simulink model "Vadim"  (R2022a)
settings: Solver=FixedStepDiscrete  StartTime=0.0  StopTime=Time*9360  RelTol=1e-3
InitFcn:
  | Time = 40;
  | PowerDelay = Time*100;
values from neighbouring files (symbols this model uses):
  a = 0.0001    [Vadim.m]
  alpha = 0.4    [Vadim.m]
  R = 10    [Vadim.m]
libraries: sim_stud_lib_r2022a x5, dspsrcs4 x2, dspsigops x2, dspswit3 x1
settings Model: Creator=RolePups  LastModifiedBy=RolePups

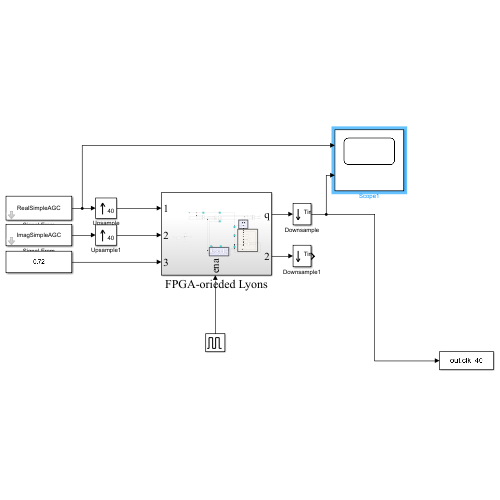
[thumbnail: Simulink's stored preview of the top-level diagram]
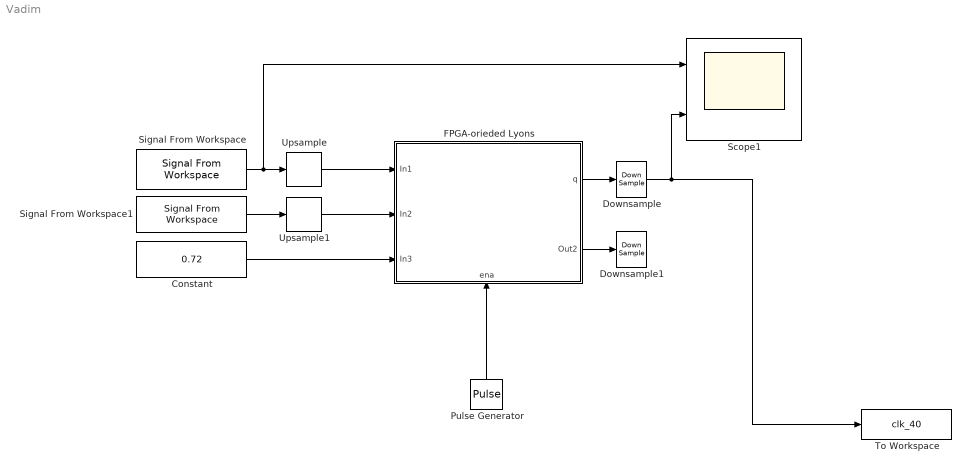
== system Vadim ==
  Constant : Constant  Value=0.72
  Downsample : DownSample  N=Time  RateOptions=Allow multirate processing
  Downsample1 : DownSample  N=Time  RateOptions=Allow multirate processing
  FPGA-orieded Lyons : Subsystem
      settings: PortSchema="{\"entries\":[{\"content\":{\"sides\":[{\"content\":{\"connectorIds\":[\"In1\",\"In2\",\"In3\"]},\"type\":\"ConnectorPlacement.EquallySpacedRectSide\",\"uuid\":\"2382ef4f-8b23-4fd9-9999-ae4ff3838c30\"},{\"content\":{\"connectorIds\":[\"Out1\",\"Out2\"],\"side\":\"RIGHT\"},\"type\":\"ConnectorPlacement.EquallySpacedRectSide\",\"uuid\":\"ff744322-ad90-46d9-948c-0637f52c7b9c\"},{\"content\":{\"connectorIds\":[],\"side\":\"TOP\"},\"type\":\"ConnectorPlacement.EquallySpacedRectSide\",\"uuid\":\"b0276f26-9e78-4e39-abf6-7a1348b88309\"},{\"content\":{\"connectorIds\":[\"In4\"],\"side\":\"BOTTOM\"},\"type\":\"ConnectorPlacement.EquallySpacedRectSide\",\"uuid\":\"b0dd70ff-8907-4b14-a46e-e3bbf4bdcae4\"}]},\"type\":\"ConnectorPlacement.EquallySpacedConnector\",\"uuid\":\"3f5cde89-4d4f-4bf7-b554-70cc79020603\"}],\"packageUris\":[\"http://schema.mathworks.com/mf0/Connector/R2020b\"],\"version\":\"1.0\"}"
  Pulse Generator : DiscretePulseGenerator  PulseType=Time based  Period=Time  PulseWidth=1/Time*100
  Scope1 : Scope  NumInputPorts=2
  Signal From Workspace : dspsrcs4/Signal From Workspace  X=RealSimpleAGC  Ts=Time  nsamps=1  OutputAfterFinalValue=Setting to zero  ignoreOrWarnInputAndFrameLengths=off  OutputFrames=off
  Signal From Workspace1 : dspsrcs4/Signal From Workspace  X=ImagSimpleAGC  Ts=Time  nsamps=1  OutputAfterFinalValue=Setting to zero  ignoreOrWarnInputAndFrameLengths=off  OutputFrames=off
  To Workspace : ToWorkspace  VariableName=clk_40  SampleTime=-1
  Upsample : dspsigops/Upsample  N=Time  phase=0  RateOptions=Allow multirate processing  ic=0  mode=Unused parameter value
  Upsample1 : dspsigops/Upsample  N=Time  phase=0  RateOptions=Allow multirate processing  ic=0  mode=Unused parameter value
  wires:
  Signal From Workspace/1 -> Scope1/1, Upsample/1
  Signal From Workspace1/1 -> Upsample1/1
  Upsample1/1 -> FPGA-orieded Lyons/2(In2)
  Constant/1 -> FPGA-orieded Lyons/3(In3)
  Pulse Generator/1 -> FPGA-orieded Lyons/4(ena)
  Upsample/1 -> FPGA-orieded Lyons/1(In1)
  FPGA-orieded Lyons/1(q) -> Downsample/1
  Downsample/1 -> Scope1/2, To Workspace/1
  FPGA-orieded Lyons/2(Out2) -> Downsample1/1

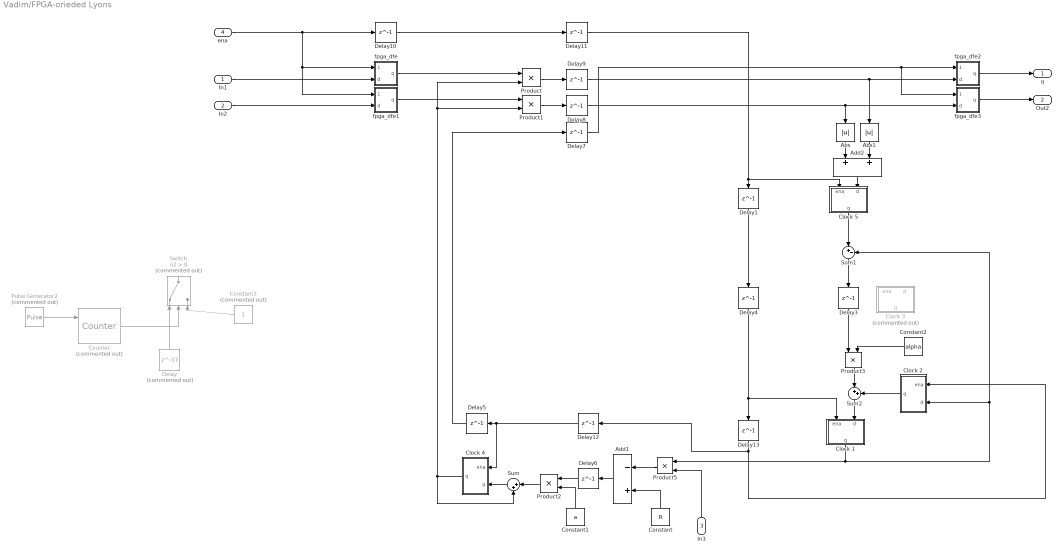
== system Vadim/FPGA-orieded Lyons ==
  In1 : Inport
  In2 : Inport  Port=2
  In3 : Inport  Port=3
  ena : Inport  Port=4
  Abs : Abs  SaturateOnIntegerOverflow=off
  Abs1 : Abs  SaturateOnIntegerOverflow=off
  Add1 : Sum  Inputs=-+  AccumDataTypeStr=double
  Add2 : Sum  AccumDataTypeStr=double
  Clock 1 : Subsystem
  Clock 2 : Subsystem
  Clock 3 : Subsystem  Commented=on
  Clock 4 : Subsystem
  Clock 5 : Subsystem
  Constant : Constant  Value=R  SampleTime=-1
  Constant1 : Constant  Value=a  SampleTime=-1
  Constant2 : Constant  Value=alpha  SampleTime=-1
  Constant3 : Constant  Commented=on  SampleTime=-1
  Counter : dspswit3/Counter  Commented=on  Direction=Up  CountEvent=Rising edge  CounterSize=User defined  MaxCount=1  InitialCount=0  Output=Count  HitValue=32  ResetInput=on  SamplesPerFrame=1  Ts=1  CntDtype=double  HitDtype=Logical
  Delay : Delay  Commented=on  DelayLength=37  InitialCondition=0
  Delay{1,3..13} (12 alike) : Delay  DelayLength=1  InitialCondition=0
  Product{,1..3,5} (5 alike) : Product  OutDataTypeStr=double
  Pulse Generator2 : DiscretePulseGenerator  Commented=on  PulseType=Time based  Period=Time*20000  PulseWidth=50  PhaseDelay=41
  Sum : Sum  Inputs=|++  AccumDataTypeStr=double
  Sum1 : Sum  Inputs=|+-  AccumDataTypeStr=double
  Sum2 : Sum  Inputs=|++  AccumDataTypeStr=double
  Switch : Switch  Commented=on  Criteria=u2 > Threshold  SaturateOnIntegerOverflow=off  InputSameDT=off
  fpga_dfe : Subsystem  AncestorBlock=sim_stud_lib_r2022a/fpga_dfe
      mask Display:
      | disp('D');
      | port_label('input',1,'e');
      | port_label('input',2,'d');
      | port_label('output',1,'q');
  fpga_dfe1 : Subsystem  AncestorBlock=sim_stud_lib_r2022a/fpga_dfe
      mask Display:
      | disp('D');
      | port_label('input',1,'e');
      | port_label('input',2,'d');
      | port_label('output',1,'q');
  fpga_dfe2 : Subsystem  AncestorBlock=sim_stud_lib_r2022a/fpga_dfe
      mask Display:
      | disp('D');
      | port_label('input',1,'e');
      | port_label('input',2,'d');
      | port_label('output',1,'q');
  fpga_dfe3 : Subsystem  AncestorBlock=sim_stud_lib_r2022a/fpga_dfe
      mask Display:
      | disp('D');
      | port_label('input',1,'e');
      | port_label('input',2,'d');
      | port_label('output',1,'q');
  q : Outport
  Out2 : Outport  Port=2
  wires:
  Clock 4/1(q) -> Sum/2, Product1/2, Product/2
  Product/1 -> Delay9/1
  Product1/1 -> Delay8/1
  Constant/1 -> Add1/2
  Sum/1 -> Clock 4/2(d)
  Product2/1 -> Sum/1
  Constant1/1 -> Product2/2
  Abs1/1 -> Add2/2
  Abs/1 -> Add2/1
  In3/1 -> Product5/2
  Product5/1 -> Add1/1
  Constant2/1 -> Product3/2
  Product3/1 -> Sum2/1
  Clock 2/1(q) -> Sum2/2
  fpga_dfe/1(q) -> Product/1
  fpga_dfe1/1(q) -> Product1/1
  Add1/1 -> Delay6/1
  Constant3/1 -> Switch/3
  Counter/1 -> Switch/2
  Pulse Generator2/1 -> Counter/1
  Sum2/1 -> Clock 1/2(d)
  Clock 1/1(q) -> Product5/1, Sum1/2, Clock 2/2(d)
  Delay/1 -> Switch/1
  fpga_dfe2/1(q) -> q/1
  fpga_dfe3/1(q) -> Out2/1
  Add2/1 -> Clock 5/2(d)
  Clock 5/1(q) -> Sum1/1
  In1/1 -> fpga_dfe/2(d)
  In2/1 -> fpga_dfe1/2(d)
  Delay8/1 -> fpga_dfe3/2(d), Abs/1
  Delay9/1 -> Abs1/1, fpga_dfe2/2(d)
  Sum1/1 -> Delay3/1
  Delay3/1 -> Product3/1
  Delay4/1 -> Delay13/1, Clock 1/1(ena)
  Delay13/1 -> Clock 2/1(ena), Delay12/1
  Delay6/1 -> Product2/1
  Delay5/1 -> Delay7/1
  Delay7/1 -> fpga_dfe3/1(ena), fpga_dfe2/1(ena)
  ena/1 -> Delay10/1, fpga_dfe1/1(ena), fpga_dfe/1(ena)
  Delay10/1 -> Delay11/1
  Delay11/1 -> Clock 5/1(ena), Delay1/1
  Delay1/1 -> Delay4/1
  Delay12/1 -> Clock 4/1(ena), Delay5/1

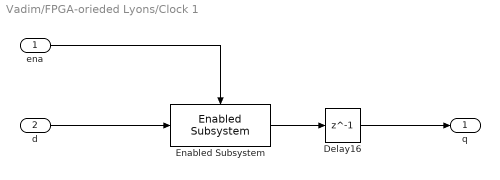
== system Vadim/FPGA-orieded Lyons/Clock 1 ==
  ena : Inport
  d : Inport  Port=2
  Delay16 : Delay  DelayLength=1
  Enabled Subsystem : sim_stud_lib_r2022a/fpga_dfe/Enabled Subsystem  SystemSampleTime=-1  VariantActivationTime=update diagram  Latency=0  AutoFrameSizeCalculation=off
  q : Outport  VectorParamsAs1DForOutWhenUnconnected=off
  wires:
  Delay16/1 -> q/1
  d/1 -> Enabled Subsystem/1
  Enabled Subsystem/1 -> Delay16/1
  ena/1 -> Enabled Subsystem/Enable

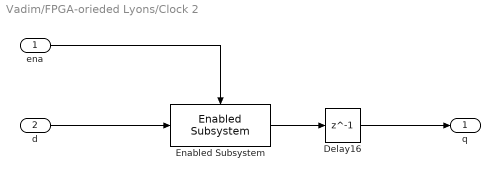
== system Vadim/FPGA-orieded Lyons/Clock 2 ==
  ena : Inport
  d : Inport  Port=2
  Delay16 : Delay  DelayLength=1
  Enabled Subsystem : sim_stud_lib_r2022a/fpga_dfe/Enabled Subsystem  SystemSampleTime=-1  VariantActivationTime=update diagram  Latency=0  AutoFrameSizeCalculation=off
  q : Outport  VectorParamsAs1DForOutWhenUnconnected=off
  wires:
  Delay16/1 -> q/1
  d/1 -> Enabled Subsystem/1
  Enabled Subsystem/1 -> Delay16/1
  ena/1 -> Enabled Subsystem/Enable

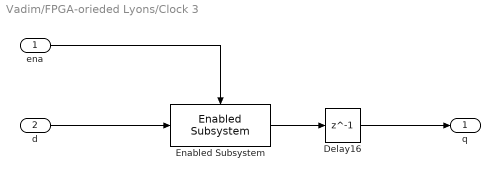
== system Vadim/FPGA-orieded Lyons/Clock 3 ==
  ena : Inport
  d : Inport  Port=2
  Delay16 : Delay  DelayLength=1
  Enabled Subsystem : sim_stud_lib_r2022a/fpga_dfe/Enabled Subsystem  SystemSampleTime=-1  VariantActivationTime=update diagram  Latency=0  AutoFrameSizeCalculation=off
  q : Outport  VectorParamsAs1DForOutWhenUnconnected=off
  wires:
  Delay16/1 -> q/1
  d/1 -> Enabled Subsystem/1
  Enabled Subsystem/1 -> Delay16/1
  ena/1 -> Enabled Subsystem/Enable

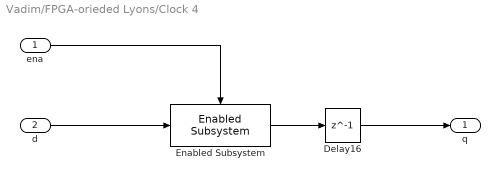
== system Vadim/FPGA-orieded Lyons/Clock 4 ==
  ena : Inport
  d : Inport  Port=2
  Delay16 : Delay  DelayLength=1
  Enabled Subsystem : sim_stud_lib_r2022a/fpga_dfe/Enabled Subsystem  SystemSampleTime=-1  VariantActivationTime=update diagram  Latency=0  AutoFrameSizeCalculation=off
  q : Outport  VectorParamsAs1DForOutWhenUnconnected=off
  wires:
  Delay16/1 -> q/1
  d/1 -> Enabled Subsystem/1
  Enabled Subsystem/1 -> Delay16/1
  ena/1 -> Enabled Subsystem/Enable

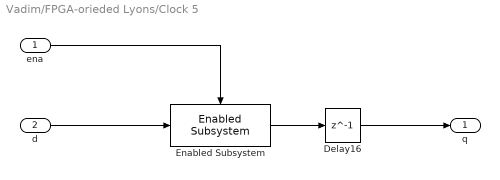
== system Vadim/FPGA-orieded Lyons/Clock 5 ==
  ena : Inport
  d : Inport  Port=2
  Delay16 : Delay  DelayLength=1
  Enabled Subsystem : sim_stud_lib_r2022a/fpga_dfe/Enabled Subsystem  SystemSampleTime=-1  VariantActivationTime=update diagram  Latency=0  AutoFrameSizeCalculation=off
  q : Outport  VectorParamsAs1DForOutWhenUnconnected=off
  wires:
  Delay16/1 -> q/1
  d/1 -> Enabled Subsystem/1
  Enabled Subsystem/1 -> Delay16/1
  ena/1 -> Enabled Subsystem/Enable

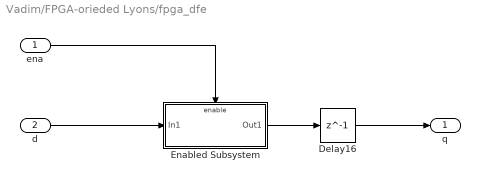
== system Vadim/FPGA-orieded Lyons/fpga_dfe ==
  ena : Inport
  d : Inport  Port=2
  Delay16 : Delay  DelayLength=1
  Enabled Subsystem : Subsystem  TreatAsAtomicUnit=on
  q : Outport  VectorParamsAs1DForOutWhenUnconnected=off
  wires:
  Enabled Subsystem/1(Out1) -> Delay16/1
  Delay16/1 -> q/1
  ena/1 -> Enabled Subsystem/Enable
  d/1 -> Enabled Subsystem/1(In1)

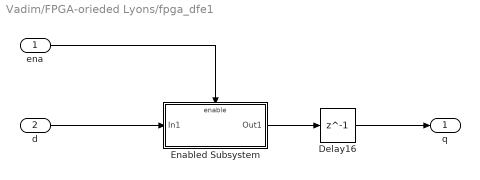
== system Vadim/FPGA-orieded Lyons/fpga_dfe1 ==
  ena : Inport
  d : Inport  Port=2
  Delay16 : Delay  DelayLength=1
  Enabled Subsystem : Subsystem  TreatAsAtomicUnit=on
  q : Outport  VectorParamsAs1DForOutWhenUnconnected=off
  wires:
  Enabled Subsystem/1(Out1) -> Delay16/1
  Delay16/1 -> q/1
  ena/1 -> Enabled Subsystem/Enable
  d/1 -> Enabled Subsystem/1(In1)

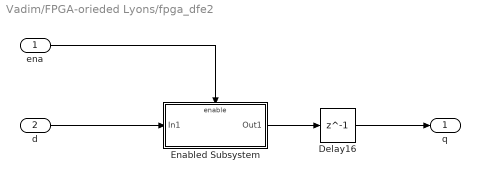
== system Vadim/FPGA-orieded Lyons/fpga_dfe2 ==
  ena : Inport
  d : Inport  Port=2
  Delay16 : Delay  DelayLength=1
  Enabled Subsystem : Subsystem  TreatAsAtomicUnit=on
  q : Outport  VectorParamsAs1DForOutWhenUnconnected=off
  wires:
  Enabled Subsystem/1(Out1) -> Delay16/1
  Delay16/1 -> q/1
  ena/1 -> Enabled Subsystem/Enable
  d/1 -> Enabled Subsystem/1(In1)

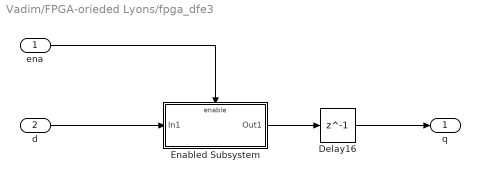
== system Vadim/FPGA-orieded Lyons/fpga_dfe3 ==
  ena : Inport
  d : Inport  Port=2
  Delay16 : Delay  DelayLength=1
  Enabled Subsystem : Subsystem  TreatAsAtomicUnit=on
  q : Outport  VectorParamsAs1DForOutWhenUnconnected=off
  wires:
  Enabled Subsystem/1(Out1) -> Delay16/1
  Delay16/1 -> q/1
  ena/1 -> Enabled Subsystem/Enable
  d/1 -> Enabled Subsystem/1(In1)

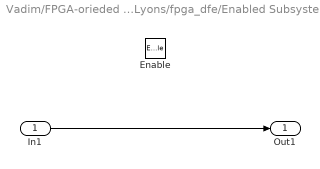
== system Vadim/FPGA-orieded Lyons/fpga_dfe/Enabled Subsystem ==
  In1 : Inport
  Enable : EnablePort
  Out1 : Outport  VectorParamsAs1DForOutWhenUnconnected=off
  wires:
  In1/1 -> Out1/1

== system Vadim/FPGA-orieded Lyons/fpga_dfe1/Enabled Subsystem ==
  In1 : Inport
  Enable : EnablePort
  Out1 : Outport  VectorParamsAs1DForOutWhenUnconnected=off
  wires:
  In1/1 -> Out1/1

== system Vadim/FPGA-orieded Lyons/fpga_dfe2/Enabled Subsystem ==
  In1 : Inport
  Enable : EnablePort
  Out1 : Outport  VectorParamsAs1DForOutWhenUnconnected=off
  wires:
  In1/1 -> Out1/1

== system Vadim/FPGA-orieded Lyons/fpga_dfe3/Enabled Subsystem ==
  In1 : Inport
  Enable : EnablePort
  Out1 : Outport  VectorParamsAs1DForOutWhenUnconnected=off
  wires:
  In1/1 -> Out1/1
